simulink model "rl"  (R2022b)
settings: Solver=VariableStepAuto  StartTime=0.0  StopTime=0.1  RelTol=1e-7
model workspace (MAT data in the model file):
  L = Simulink.Parameter
  L.Value = 0.095
  L.DataType = 'auto'
  L.Complexity = 'real'
  L.Dimensions = [1 1]
  R = 40
  a = 220
  freq = 314.16
values from neighbouring files (symbols this model uses):
  L = 0.095    [lab1.m]
settings Model: Creator=axelfroborg  LastModifiedBy=emill
settings SolverCC: AlgebraicLoopSolver=TrustRegion
settings DebuggingCC: UnconnectedInputMsg=warning  UnconnectedOutputMsg=warning  UnconnectedLineMsg=warning  SFMachineParentedDataDiag=warning
settings ModelReferenceCC: EnableRefExpFcnMdlSchedulingChecks=on
settings RTWCC: DLArmComputeVersion=19.05

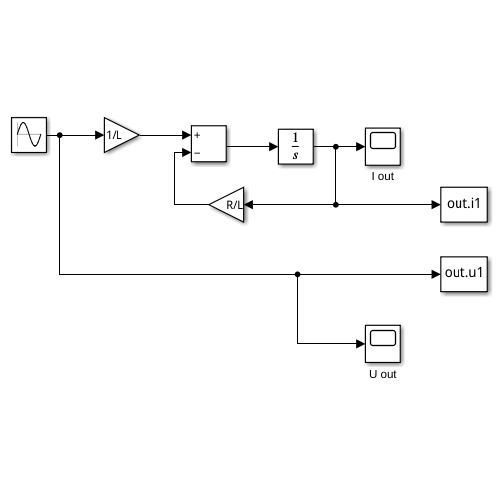
[thumbnail: Simulink's stored preview of the top-level diagram]
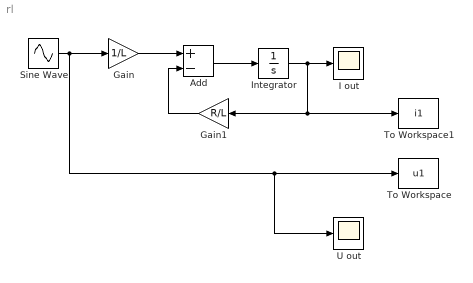
== system rl ==
  Add : Sum  Inputs=+-
  Gain : Gain  Gain=1/L
  Gain1 : Gain  Gain=R/L
  I out : Scope
  Integrator : Integrator
  Sine Wave : Sin  Amplitude=220  Frequency=freq  SampleTime=0
  To Workspace : ToWorkspace  VariableName=u1  SampleTime=-1
  To Workspace1 : ToWorkspace  VariableName=i1  SampleTime=-1
  U out : Scope
  wires:
  Integrator/1 -> Gain1/1, To Workspace1/1, I out/1
  Gain1/1 -> Add/2
  Sine Wave/1 -> Gain/1, U out/1, To Workspace/1
  Gain/1 -> Add/1
  Add/1 -> Integrator/1
